simulink model "TD_PITCH"  (R2019b)
settings: Solver=VariableStepAuto  StartTime=0.0  StopTime=10.0  RelTol=1e-3
undefined symbols (not defined in the file): Dm, Dt, g, Jeq, k_pitch_, Mb
settings Model: Creator=lbend  LastModifiedBy=lbend

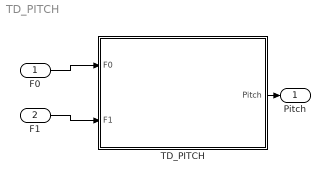
== system TD_PITCH ==
  F0 : Inport
  "F1 " : Inport  Port=2
  TD_PITCH : Subsystem
  Pitch : Outport
  wires:
  F0/1 -> TD_PITCH/1(F0)
  "F1 "/1 -> TD_PITCH/2("F1 ")
  TD_PITCH/1(Pitch) -> Pitch/1

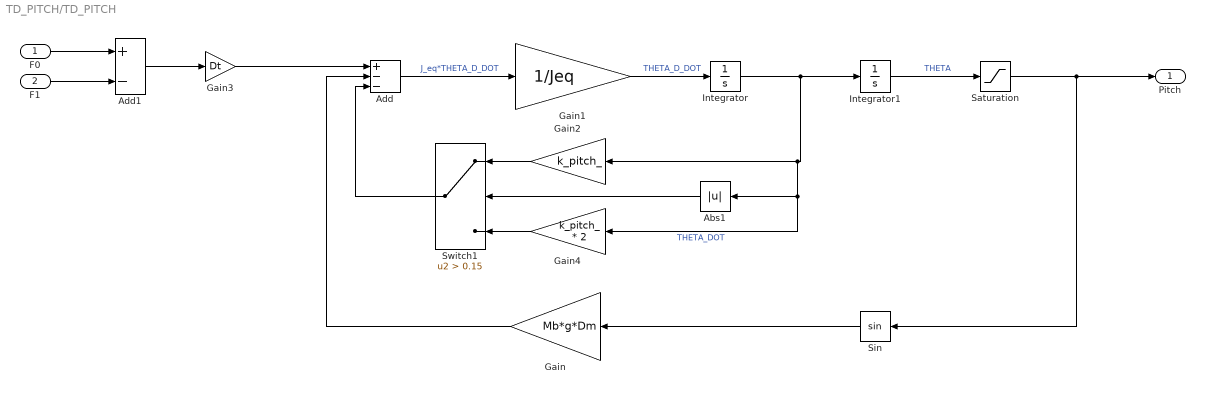
== system TD_PITCH/TD_PITCH ==
  F0 : Inport
  "F1 " : Inport  Port=2
  Abs1 : Abs
  Add : Sum  Inputs=+--
  Add1 : Sum  Inputs=+-
  Gain : Gain  Gain=Mb*g*Dm
  Gain1 : Gain  Gain=1/Jeq
  Gain2 : Gain  Gain=k_pitch_
  Gain3 : Gain  Gain=Dt
  Gain4 : Gain  Gain=k_pitch_ * 2
  Integrator : Integrator
  Integrator1 : Integrator
  Saturation : Saturate  UpperLimit=0.93  LowerLimit=-0.93
  Sin : Trigonometry
  Switch1 : Switch  Criteria=u2 > Threshold  Threshold=0.15
  Pitch : Outport
  wires:
  Integrator/1 -> Gain2/1, Gain4/1, Abs1/1, Integrator1/1  "THETA_DOT"
  Gain3/1 -> Add/1
  "F1 "/1 -> Add1/2
  Add1/1 -> Gain3/1
  Saturation/1 -> Pitch/1, Sin/1
  Gain1/1 -> Integrator/1  "THETA_D_DOT"
  Integrator1/1 -> Saturation/1  "THETA"
  Gain/1 -> Add/2
  Abs1/1 -> Switch1/2
  Switch1/1 -> Add/3
  Sin/1 -> Gain/1
  F0/1 -> Add1/1
  Add/1 -> Gain1/1  "J_eq*THETA_D_DOT"
  Gain4/1 -> Switch1/3
  Gain2/1 -> Switch1/1
